simulink model "TestUSART_Rcv_Send_SIT"  (R2015b)
settings: Solver=FixedStepDiscrete  StartTime=0.0  StopTime=10.0  RelTol=1e-3
libraries: GPIO_Lib x2, USART_Lib x2, STM32_Config_Lib x1
settings Model: Creator=reynaudp  LastModifiedBy=reynaudp
settings DataIOCC: SaveFormat=Array  SignalLoggingSaveFormat=ModelDataLogs
settings OptimizationCC: OptimizeModelRefInitCode=on  LifeSpan=1
settings DebuggingCC: UnderspecifiedInitializationDetection=Classic  MergeDetectMultiDrivingBlocksExec=none  SolverPrmCheckMsg=warning  MultiTaskDSMMsg=warning  MultiTaskCondExecSysMsg=none
settings HardwareCC: ProdBitPerPointer=32  ProdLargestAtomicInteger=Integer  ProdWordSize=32  ProdHWDeviceType=STMicroelectronics->STM32 32-bit Cortex-M
settings RTWCC: SystemTargetFile=stm32.tlc  TemplateMakefile=stm32.tmf  Description=stm32 (Embedded Target)  GenerateReport=on  LaunchReport=on
settings CodeAppCC: IgnoreCustomStorageClasses=off  MaxIdLength=64  CustomSymbolStrType=$N$R$M  SimulinkBlockComments=off
settings STFCustomTargetCC: CodeReplacementLibrary=ARM CMSIS SIN COS  ParMdlRefBuildCompliant=on  ConcurrentExecutionCompliant=off  IncludeMdlTerminateFcn=off  GeneratePreprocessorConditionals=Use local settings  CombineOutputUpdateFcns=on  ERTCustomFileBanners=on  SupportContinuousTime=off  SupportNonInlinedSFcns=off  SupportVariableSizeSignals=on  MATLABClassNameForMDSCustomization=Simulink.SoftwareTarget.ERTCustomization  CPPClassGenCompliant=off  GRTInterface=off  SystemTargetFile=stm32.tlc
settings ERTTargetCC: CodeReplacementLibrary=ARM CMSIS SIN COS  CompOptLevelCompliant=off  ConcurrentExecutionCompliant=off  IncludeMdlTerminateFcn=off  ERTFirstTimeCompliant=off  SupportVariableSizeSignals=on  ModelStepFunctionPrototypeControlCompliant=off  CPPClassGenCompliant=off  UseToolchainInfoCompliant=off  ERTSrcFileBannerTemplate=sourceFileTemplate.cgt  ERTHdrFileBannerTemplate=sourceFileTemplate.cgt  ERTDataSrcFileTemplate=sourceFileTemplate.cgt  ERTDataHdrFileTemplate=sourceFileTemplate.cgt  ERTCustomFileTemplate=customRoutineProcess.tlc
settings ConfigComp: CovModelRefEnable=Off  CovSFcnEnable=off

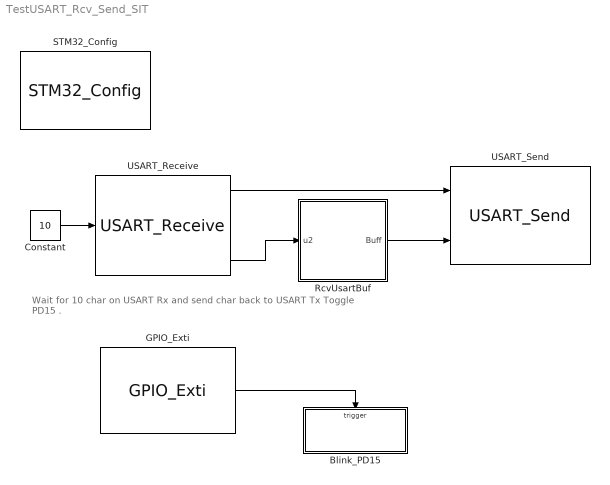
== system TestUSART_Rcv_Send_SIT ==
  note: Wait for 10 char on USART Rx and send char back to USART Tx
      | Toggle PD15 .
  Blink_PD15 : Subsystem  TreatAsAtomicUnit=on
  Constant : Constant  Value=10  OutDataTypeStr=uint16
  GPIO_Exti : GPIO_Lib/GPIO_Exti  Port_name=GPIOA  Pin_0=on  Pin_1=off  Pin_2=off  Pin_3=off  Pin_4=off  Pin_5=off  Pin_6=off  Pin_7=off  Pin_8=off  Pin_9=off  Pin_10=off  Pin_11=off  Pin_12=off  Pin_13=off  Pin_14=off  Pin_15=off  PinList=GPIOA0
  RcvUsartBuf : MATLAB Function  TreatAsAtomicUnit=on
  STM32_Config : STM32_Config_Lib/STM32_Config  Priority=0  Project_Path=.\  Config_File=TestUSART_Rcv_Send_SIT.ioc  MCU_Name=STM32F407VGTx
  USART_Receive : USART_Lib/USART_Receive  USART_name=USART1  Buff_size=32  nbUsart=1  Soft_it=on  Soft_num=0  usartMode=Asynchronous  usartDma_Rx=on  usartDma_Tx=on  usartIt=on
  USART_Send : USART_Lib/USART_Send  USART_name=USART1  Buff_size=32  nbUsart=1  usartMode=Asynchronous  usartDma_Rx=on  usartDma_Tx=on  usartIt=on
  wires:
  Constant/1 -> USART_Receive/1
  GPIO_Exti/1 -> Blink_PD15/Trigger
  RcvUsartBuf/1(Buff) -> USART_Send/2
  USART_Receive/3 -> RcvUsartBuf/1(u2)
  USART_Receive/1 -> USART_Send/1

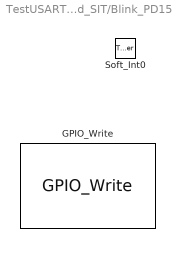
== system TestUSART_Rcv_Send_SIT/Blink_PD15 ==
  Soft_Int0 : TriggerPort  TriggerType=function-call
  GPIO_Write : GPIO_Lib/GPIO_Write  Port_name=GPIOD  Pin0=off  Toggle_Pin0=off  Pin1=off  Toggle_Pin1=off  Pin2=off  Toggle_Pin2=off  Pin3=off  Toggle_Pin3=off  Pin4=off  Toggle_Pin4=off  Pin5=off  Toggle_Pin5=off  Pin6=off  Toggle_Pin6=off  Pin7=off  Toggle_Pin7=off  Pin8=off  Toggle_Pin8=off  Pin9=off  Toggle_Pin9=off  Pin10=off  Toggle_Pin10=off  Pin11=off  Toggle_Pin11=off  Pin12=off  Toggle_Pin12=off  Pin13=off  Toggle_Pin13=off  Pin14=off  Toggle_Pin14=off  Pin15=on  Toggle_Pin15=on  PinList=GPIOD15

== matlab function TestUSART_Rcv_Send_SIT/RcvUsartBuf ==
  data: Buff output uint32 size=1; u2 input
function Buff = convert(u2)
if coder.target('Sfun')
% Executing in MATLAB, Buff is null
Buff = uint32(0);
%NbChar = uint16(0);
else
% Executing in the generated code. 
%CH1Msg = zeros(1,u1 + 3,'uint8');
%coder.ceval('strncpy',coder.wref(CH1Msg),u2,u1);
%CH1Msg = [CH1Msg, 13, 10, 0];
Buff = coder.ceval('getBuffPtr',coder.ref(u2));
%NbChar = coder.ceval('strlen',coder.wref(u2));
end
end
